simulink model "hdmpc_pns_cstr"  (Simulink 8.8)
settings: Solver=ode45  StartTime=0  StopTime=Tsim  RelTol=1e-3  EnableMultiTasking=on
values from neighbouring files (symbols this model uses):
  SubsystemMPC =     [agent.mat]
undefined symbols (not defined in the file or in its folder): Ac, Bc, Cc, Dc, HDMPC, hdmpc_control, Lc
settings Model: Creator=stefano  LastModifiedBy=trinhvv-admin
settings DataIOCC: SaveOutput=off  SignalLogging=off  DSMLogging=off  SaveTime=off
settings OptimizationCC: ExpressionDepthLimit=2147483647

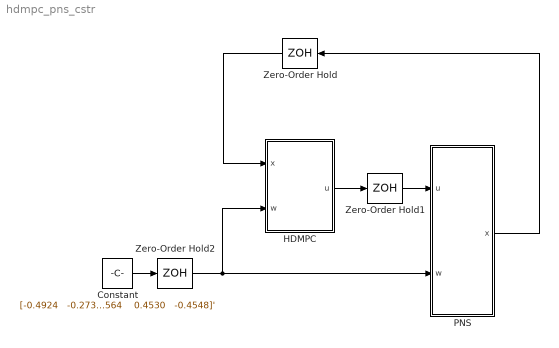
== system hdmpc_pns_cstr ==
  Constant : Constant  Value="[-0.4924   -0.2739   -0.2564    0.4530   -0.4548]'"
  HDMPC : Subsystem
  PNS : Subsystem
  Zero-Order Hold : ZeroOrderHold
  Zero-Order Hold1 : ZeroOrderHold
  Zero-Order Hold2 : ZeroOrderHold
  wires:
  PNS/1(x) -> Zero-Order Hold/1
  Constant/1 -> Zero-Order Hold2/1
  Zero-Order Hold/1 -> HDMPC/1(x)
  Zero-Order Hold1/1 -> PNS/1(u)
  HDMPC/1(u) -> Zero-Order Hold1/1
  Zero-Order Hold2/1 -> PNS/2(w), HDMPC/2(w)

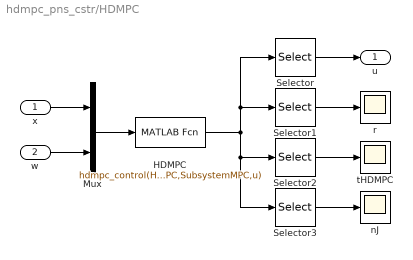
== system hdmpc_pns_cstr/HDMPC ==
  x : Inport
  w : Inport  Port=2
  HDMPC : MATLABFcn  MATLABFcn=hdmpc_control(HDMPC,SubsystemMPC,u)  OutputDimensions=12
  Mux : Mux  Inputs=2
  Selector : Selector  IndexOptions=Index vector (dialog)  Indices=1:5  OutputSizes=1
  Selector1 : Selector  IndexOptions=Index vector (dialog)  Indices=6:10  OutputSizes=1
  Selector2 : Selector  IndexOptions=Index vector (dialog)  Indices=11  OutputSizes=1
  Selector3 : Selector  IndexOptions=Index vector (dialog)  Indices=12  OutputSizes=1
  nJ : Scope
  r : Scope
  tHDMPC : Scope
  u : Outport
  wires:
  Selector/1 -> u/1
  HDMPC/1 -> Selector3/1, Selector2/1, Selector/1, Selector1/1
  Mux/1 -> HDMPC/1
  x/1 -> Mux/1
  w/1 -> Mux/2
  Selector1/1 -> r/1
  Selector2/1 -> tHDMPC/1
  Selector3/1 -> nJ/1

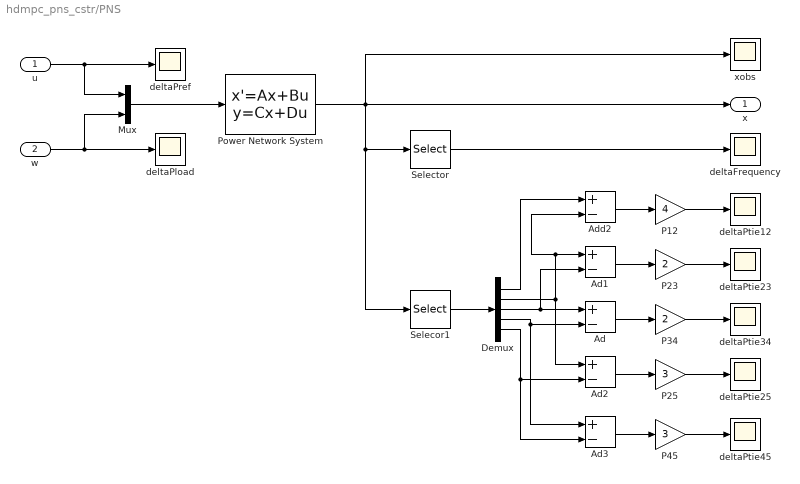
== system hdmpc_pns_cstr/PNS ==
  u : Inport
  w : Inport  Port=2
  Ad{,1..3} (4 alike) : Sum  Inputs=+-
  Add2 : Sum  Inputs=+-
  Demux : Demux  Outputs=5
  Mux : Mux  Inputs=2
  P12 : Gain  Gain=4
  P23 : Gain  Gain=2
  P25 : Gain  Gain=3
  P34 : Gain  Gain=2
  P45 : Gain  Gain=3
  Power Network System : StateSpace  A=Ac  B=[ Bc Lc ]  C=Cc  D=[ Dc zeros(size(Cc,1),size(Lc,2)) ]  X0=|
      | [    0.1278
      |     0.1216
      |    -0.0778
      |    -0.0587
      |    -0.0285
      |     0.1303
      |     0.0637
      |    -0.1353
      |     0.1331
      |     0.1492
      |    -0.1494
      |    -0.1586
      |     0.0766
      |    -0.1775
      |    -0.0478
      |    -0.0889
      |    -0.0121
      |     0.1802
      |     0.0014
      |     0.0797]'
  Selecor1 : Selector  InputPortWidth=20  IndexOptions=Index vector (dialog)  Indices=1:4:size(Ac,1)  OutputSizes=1
  Selector : Selector  InputPortWidth=20  IndexOptions=Index vector (dialog)  Indices=2:4:size(Ac,1)  OutputSizes=1
  deltaFrequency : Scope
  deltaPload : Scope
  deltaPref : Scope
  deltaPtie{12,23,25,34,45} (5 alike) : Scope
  xobs : Scope
  x : Outport
  wires:
  Mux/1 -> Power Network System/1
  w/1 -> Mux/2, deltaPload/1
  u/1 -> Mux/1, deltaPref/1
  Power Network System/1 -> x/1, Selecor1/1, Selector/1, xobs/1
  Selector/1 -> deltaFrequency/1
  Selecor1/1 -> Demux/1
  Add2/1 -> P12/1
  P12/1 -> deltaPtie12/1
  Ad1/1 -> P23/1
  P23/1 -> deltaPtie23/1
  Ad/1 -> P34/1
  P34/1 -> deltaPtie34/1
  Demux/1 -> Add2/1
  Demux/2 -> Add2/2, Ad1/1, Ad2/1
  Demux/3 -> Ad1/2, Ad/1
  Demux/4 -> Ad3/1, Ad/2
  Ad2/1 -> P25/1
  P25/1 -> deltaPtie25/1
  Ad3/1 -> P45/1
  P45/1 -> deltaPtie45/1
  Demux/5 -> Ad3/2, Ad2/2
